simulink library "controls_module_lib"  (R2024b)
settings: Solver=VariableStepAuto  StartTime=0.0  StopTime=10.0  RelTol=1e-3
undefined symbols (not defined in the file): j, S_NOM, SNOM, VLL, VLL_NOM
libraries: simulink x14
(part 2 of 2)

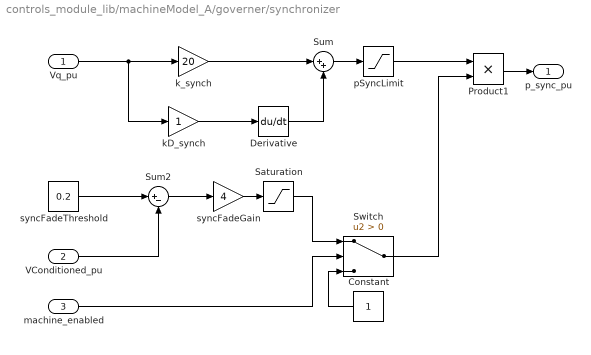
== system controls_module_lib/machineModel_A/governer/synchronizer ==
  Vq_pu : Inport
  VConditioned_pu : Inport  Port=2
  machine_enabled : Inport  Port=3
  Constant : Constant
  Derivative : Derivative
  Product1 : Product
  Saturation : Saturate  UpperLimit=1  LowerLimit=0
  Sum : Sum  Inputs=|++
  Sum2 : Sum  Inputs=|+-
  Switch : Switch  Criteria=u2 > Threshold  SaturateOnIntegerOverflow=off  InputSameDT=off
  kD_synch : Gain
  k_synch : Gain  Gain=20
  pSyncLimit : Saturate  UpperLimit=3  LowerLimit=-3
  syncFadeGain : Gain  Gain=4
  syncFadeThreshold : Constant  Value=0.2
  p_sync_pu : Outport
  wires:
  Vq_pu/1 -> kD_synch/1, k_synch/1
  Switch/1 -> Product1/2
  syncFadeThreshold/1 -> Sum2/1
  Saturation/1 -> Switch/1
  syncFadeGain/1 -> Saturation/1
  machine_enabled/1 -> Switch/2
  Sum2/1 -> syncFadeGain/1
  VConditioned_pu/1 -> Sum2/2
  Constant/1 -> Switch/3
  Product1/1 -> p_sync_pu/1
  Sum/1 -> pSyncLimit/1
  k_synch/1 -> Sum/1
  Derivative/1 -> Sum/2
  kD_synch/1 -> Derivative/1
  pSyncLimit/1 -> Product1/1

== system controls_module_lib/machineModel_A/rotor model/oscillator_3ph ==
  f : Inport
  Cos : Trigonometry  Operator=cos
  Gain : Gain  Gain=2*pi
  Integrator : Integrator
  Real-Imag to Complex : RealImagToComplex
  Sin : Trigonometry
  Sum1 : Sum  Inputs=|++
  phase_shift : Constant  Value=[0 -1/3 -2/3]
  osc[3] : Outport
  wires:
  Sum1/1 -> Gain/1
  phase_shift/1 -> Sum1/2
  Sin/1 -> Real-Imag to Complex/2
  Integrator/1 -> Sum1/1
  Gain/1 -> Sin/1, Cos/1
  Cos/1 -> Real-Imag to Complex/1
  Real-Imag to Complex/1 -> osc[3]/1
  f/1 -> Integrator/1
